simulink model "pet_integration_architecture"  (R2024a)
settings: Solver=FixedStepDiscrete  StartTime=0.0  StopTime=10.0  RelTol=1e-3
undefined symbols (not defined in the file or in its folder): D1, P
undefined symbols (not defined in the file): orig
(part 1 of 3)
settings Model: DataDictionary=pet_integration_data_dictionary.sldd  Creator=diell  LastModifiedBy=diell

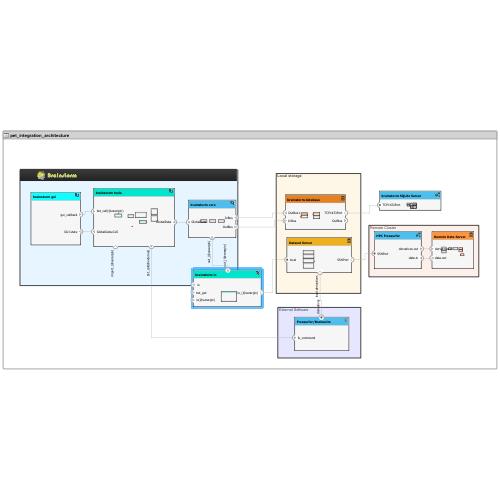
[thumbnail: Simulink's stored preview of the top-level diagram]
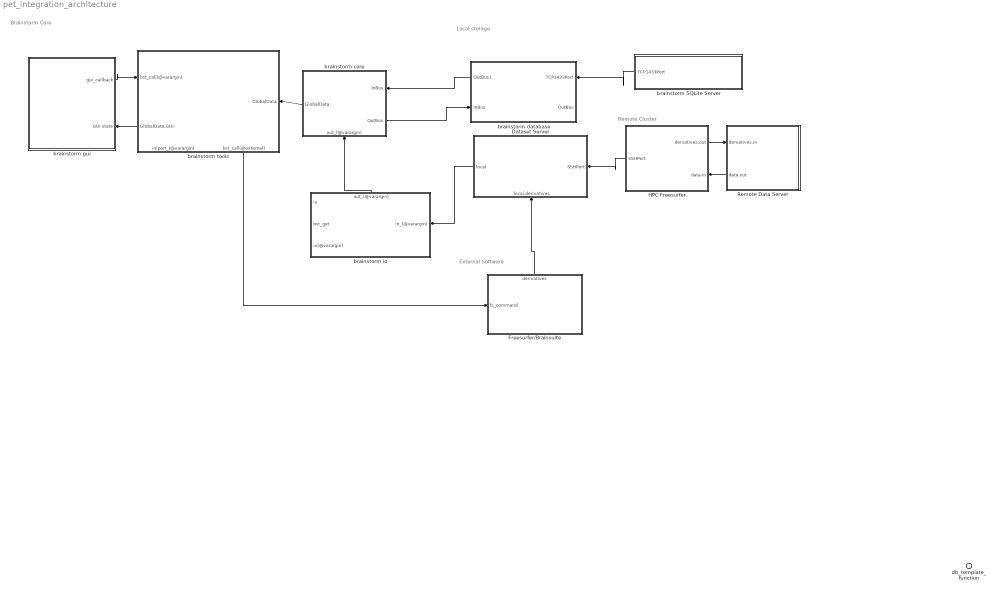
== system pet_integration_architecture ==
  note: External Software
  note: Local storage
  note: Remote Cluster
  note: Brainstorm Core
  db_template_function : Inport  OutputFunctionCall=on
  Dataset Server : Subsystem
      settings: PortSchema="{\"entries\":[{\"content\":{\"headerSize\":26,\"margin\":15,\"minimumSpacing\":25,\"sides\":[{\"content\":{\"connectorIds\":[\"Out1\"]},\"type\":\"ConnectorPlacement.EquallySpacedRectSide\",\"uuid\":\"a3539b9a-22db-4da3-b271-35b287ced3a1\"},{\"content\":{\"connectorIds\":[\"In2\"],\"side\":\"RIGHT\"},\"type\":\"ConnectorPlacement.EquallySpacedRectSide\",\"uuid\":\"72d9f298-5062-46d4-b3c5-f2fa85d7a7a6\"},{\"content\":{\"side\":\"TOP\"},\"type\":\"ConnectorPlacement.EquallySpacedRectSide\",\"uuid\":\"050469fd-3881-4b53-a813-94df038aa659\"},{\"content\":{\"connectorIds\":[\"In1\"],\"side\":\"BOTTOM\"},\"type\":\"ConnectorPlacement.EquallySpacedRectSide\",\"uuid\":\"33e80db7-af60-43f6-9c88-147327e21178\"}]},\"type\":\"ConnectorPlacement.EquallySpacedConnector\",\"uuid\":\"6db04dad-62f3-4987-a6a9-d236db4fe2a3\"}],\"packageUris\":[\"http://schema.mathworks.com/mf0/Connector/R2020b\"],\"version\":\"1.0\"}"
  Freesurfer/Brainsuite : Subsystem
      settings: PortSchema="{\"entries\":[{\"content\":{\"headerSize\":26,\"margin\":15,\"minimumSpacing\":25,\"sides\":[{\"content\":{\"connectorIds\":[\"In1\"]},\"type\":\"ConnectorPlacement.EquallySpacedRectSide\",\"uuid\":\"d9face5b-155e-4e83-95c0-d581b737b6e3\"},{\"content\":{\"side\":\"RIGHT\"},\"type\":\"ConnectorPlacement.EquallySpacedRectSide\",\"uuid\":\"f965be1f-1639-4140-b9ea-f5e9efbe4150\"},{\"content\":{\"connectorIds\":[\"Out1\"],\"side\":\"TOP\"},\"type\":\"ConnectorPlacement.EquallySpacedRectSide\",\"uuid\":\"7c9c4b2b-011c-4482-afab-b6e67025a5e2\"},{\"content\":{\"side\":\"BOTTOM\"},\"type\":\"ConnectorPlacement.EquallySpacedRectSide\",\"uuid\":\"80c85d3d-f594-4aa0-8d78-457d560265ec\"}]},\"type\":\"ConnectorPlacement.EquallySpacedConnector\",\"uuid\":\"ec963004-117d-4f22-bb00-71f35201e6e2\"}],\"packageUris\":[\"http://schema.mathworks.com/mf0/Connector/R2020b\"],\"version\":\"1.0\"}"
  HPC Freesurfer : Subsystem
      settings: PortSchema="{\"entries\":[{\"content\":{\"headerSize\":26,\"margin\":15,\"minimumSpacing\":25,\"sides\":[{\"content\":{\"connectorIds\":[\"Out1\"]},\"type\":\"ConnectorPlacement.EquallySpacedRectSide\",\"uuid\":\"d9face5b-155e-4e83-95c0-d581b737b6e3\"},{\"content\":{\"connectorIds\":[\"Out2\",\"In1\"],\"side\":\"RIGHT\"},\"type\":\"ConnectorPlacement.EquallySpacedRectSide\",\"uuid\":\"f965be1f-1639-4140-b9ea-f5e9efbe4150\"},{\"content\":{\"side\":\"TOP\"},\"type\":\"ConnectorPlacement.EquallySpacedRectSide\",\"uuid\":\"7c9c4b2b-011c-4482-afab-b6e67025a5e2\"},{\"content\":{\"side\":\"BOTTOM\"},\"type\":\"ConnectorPlacement.EquallySpacedRectSide\",\"uuid\":\"79ceda21-0cb6-4778-9565-f8bf46316a14\"}]},\"type\":\"ConnectorPlacement.EquallySpacedConnector\",\"uuid\":\"ec963004-117d-4f22-bb00-71f35201e6e2\"}],\"packageUris\":[\"http://schema.mathworks.com/mf0/Connector/R2020b\"],\"version\":\"1.0\"}"
  Remote Data Server : Subsystem
      settings: PortSchema="{\"entries\":[{\"content\":{\"headerSize\":26,\"margin\":15,\"minimumSpacing\":25,\"sides\":[{\"content\":{\"connectorIds\":[\"In1\",\"Out1\"]},\"type\":\"ConnectorPlacement.EquallySpacedRectSide\",\"uuid\":\"a3539b9a-22db-4da3-b271-35b287ced3a1\"},{\"content\":{\"side\":\"RIGHT\"},\"type\":\"ConnectorPlacement.EquallySpacedRectSide\",\"uuid\":\"72d9f298-5062-46d4-b3c5-f2fa85d7a7a6\"},{\"content\":{\"side\":\"TOP\"},\"type\":\"ConnectorPlacement.EquallySpacedRectSide\",\"uuid\":\"050469fd-3881-4b53-a813-94df038aa659\"},{\"content\":{\"side\":\"BOTTOM\"},\"type\":\"ConnectorPlacement.EquallySpacedRectSide\",\"uuid\":\"ec20b969-1eda-4ce5-89cf-082fe7652dff\"}]},\"type\":\"ConnectorPlacement.EquallySpacedConnector\",\"uuid\":\"6db04dad-62f3-4987-a6a9-d236db4fe2a3\"}],\"packageUris\":[\"http://schema.mathworks.com/mf0/Connector/R2020b\"],\"version\":\"1.0\"}"
  brainstorm SQLite Server : Subsystem
      settings: PortSchema="{\"entries\":[{\"content\":{\"headerSize\":26,\"margin\":15,\"minimumSpacing\":25,\"sides\":[{\"content\":{\"connectorIds\":[\"Out1\"]},\"type\":\"ConnectorPlacement.EquallySpacedRectSide\",\"uuid\":\"7b7365e4-3e33-4b91-9d81-29acea824425\"},{\"content\":{\"side\":\"RIGHT\"},\"type\":\"ConnectorPlacement.EquallySpacedRectSide\",\"uuid\":\"c8185be4-14fd-4b07-9d64-196ce2484816\"},{\"content\":{\"side\":\"TOP\"},\"type\":\"ConnectorPlacement.EquallySpacedRectSide\",\"uuid\":\"601e7076-ec49-4dfd-9b03-b7765df258a0\"}]},\"type\":\"ConnectorPlacement.EquallySpacedConnector\",\"uuid\":\"02951655-a26c-45d3-8145-be6034beccc3\"}],\"packageUris\":[\"http://schema.mathworks.com/mf0/Connector/R2020b\"],\"version\":\"1.0\"}"
  brainstorm core : Subsystem
      settings: PortSchema="{\"entries\":[{\"content\":{\"headerSize\":26,\"margin\":15,\"minimumSpacing\":25,\"sides\":[{\"content\":{\"connectorIds\":[\"Out2\"]},\"type\":\"ConnectorPlacement.EquallySpacedRectSide\",\"uuid\":\"f13372f0-b9c4-4d9f-b80d-b3fcffd9ebc1\"},{\"content\":{\"connectorIds\":[\"In2\",\"Out1\"],\"side\":\"RIGHT\"},\"type\":\"ConnectorPlacement.EquallySpacedRectSide\",\"uuid\":\"7a8ed507-1a09-4737-be0e-7f469c03bf31\"},{\"content\":{\"side\":\"TOP\"},\"type\":\"ConnectorPlacement.EquallySpacedRectSide\",\"uuid\":\"dcf0e4cd-c5e5-4129-a80f-1cd05790def0\"},{\"content\":{\"connectorIds\":[\"In1\"],\"side\":\"BOTTOM\"},\"type\":\"ConnectorPlacement.EquallySpacedRectSide\",\"uuid\":\"0e961a59-0b55-4a03-a714-2fdf2294d0cf\"}]},\"type\":\"ConnectorPlacement.EquallySpacedConnector\",\"uuid\":\"218acaa3-d922-4814-a102-8c4fe12f2e05\"}],\"packageUris\":[\"http://schema.mathworks.com/mf0/Connector/R2020b\"],\"version\":\"1.0\"}"
  brainstorm database : Subsystem
      settings: PortSchema="{\"entries\":[{\"content\":{\"headerSize\":26,\"margin\":15,\"minimumSpacing\":25,\"sides\":[{\"content\":{\"connectorIds\":[\"Out1\",\"In1\"]},\"type\":\"ConnectorPlacement.EquallySpacedRectSide\",\"uuid\":\"d4370dee-db71-4a38-ba8c-347b506b3053\"},{\"content\":{\"connectorIds\":[\"In2\",\"Out2\"],\"side\":\"RIGHT\"},\"type\":\"ConnectorPlacement.EquallySpacedRectSide\",\"uuid\":\"2fab9e72-f87c-493f-bacf-77c4be84942a\"},{\"content\":{\"side\":\"TOP\"},\"type\":\"ConnectorPlacement.EquallySpacedRectSide\",\"uuid\":\"3b731ab7-bbbf-4243-a071-715f3ecb33e2\"}]},\"type\":\"ConnectorPlacement.EquallySpacedConnector\",\"uuid\":\"fffe9ba9-fa34-4948-8c6e-90e3263c9a73\"}],\"packageUris\":[\"http://schema.mathworks.com/mf0/Connector/R2020b\"],\"version\":\"1.0\"}"
  brainstorm gui : Subsystem
      settings: PortSchema="{\"entries\":[{\"content\":{\"headerSize\":26,\"margin\":15,\"minimumSpacing\":25,\"sides\":[{\"content\":{},\"type\":\"ConnectorPlacement.EquallySpacedRectSide\",\"uuid\":\"d99db108-8c8a-4010-81b2-f142fbf318f5\"},{\"content\":{\"connectorIds\":[\"Out1\",\"In1\"],\"side\":\"RIGHT\"},\"type\":\"ConnectorPlacement.EquallySpacedRectSide\",\"uuid\":\"9190d96c-22e3-4cc9-a507-8f094dc67743\"},{\"content\":{\"side\":\"TOP\"},\"type\":\"ConnectorPlacement.EquallySpacedRectSide\",\"uuid\":\"08b46875-eac1-4edb-b2eb-5598dd517a75\"},{\"content\":{\"side\":\"BOTTOM\"},\"type\":\"ConnectorPlacement.EquallySpacedRectSide\",\"uuid\":\"52ff99e9-7de1-484d-abe5-5275aa089791\"}]},\"type\":\"ConnectorPlacement.EquallySpacedConnector\",\"uuid\":\"c8d2d02b-cf5a-431f-8876-22d36c8a9b33\"}],\"packageUris\":[\"http://schema.mathworks.com/mf0/Connector/R2020b\"],\"version\":\"1.0\"}"
  brainstorm io : Subsystem
      settings: PortSchema="{\"entries\":[{\"content\":{\"headerSize\":26,\"margin\":15,\"minimumSpacing\":25,\"sides\":[{\"content\":{\"connectorIds\":[\"Out1\",\"In3\",\"In2\"]},\"type\":\"ConnectorPlacement.EquallySpacedRectSide\",\"uuid\":\"d9face5b-155e-4e83-95c0-d581b737b6e3\"},{\"content\":{\"connectorIds\":[\"In1\"],\"side\":\"RIGHT\"},\"type\":\"ConnectorPlacement.EquallySpacedRectSide\",\"uuid\":\"f965be1f-1639-4140-b9ea-f5e9efbe4150\"},{\"content\":{\"connectorIds\":[\"Out2\"],\"side\":\"TOP\"},\"type\":\"ConnectorPlacement.EquallySpacedRectSide\",\"uuid\":\"7c9c4b2b-011c-4482-afab-b6e67025a5e2\"},{\"content\":{\"side\":\"BOTTOM\"},\"type\":\"ConnectorPlacement.EquallySpacedRectSide\",\"uuid\":\"6bb6967a-39ac-45ff-9bbd-a1229cc8daf0\"}]},\"type\":\"ConnectorPlacement.EquallySpacedConnector\",\"uuid\":\"ec963004-117d-4f22-bb00-71f35201e6e2\"}],\"packageUris\":[\"http://schema.mathworks.com/mf0/Connector/R2020b\"],\"version\":\"1.0\"}"
  brainstorm tools : Subsystem
      settings: PortSchema="{\"entries\":[{\"content\":{\"headerSize\":26,\"margin\":15,\"minimumSpacing\":25,\"sides\":[{\"content\":{\"connectorIds\":[\"In3\",\"Out2\"]},\"type\":\"ConnectorPlacement.EquallySpacedRectSide\",\"uuid\":\"d9face5b-155e-4e83-95c0-d581b737b6e3\"},{\"content\":{\"connectorIds\":[\"In1\"],\"side\":\"RIGHT\"},\"type\":\"ConnectorPlacement.EquallySpacedRectSide\",\"uuid\":\"f965be1f-1639-4140-b9ea-f5e9efbe4150\"},{\"content\":{\"side\":\"TOP\"},\"type\":\"ConnectorPlacement.EquallySpacedRectSide\",\"uuid\":\"7c9c4b2b-011c-4482-afab-b6e67025a5e2\"},{\"content\":{\"connectorIds\":[\"In2\",\"Out1\"],\"side\":\"BOTTOM\"},\"type\":\"ConnectorPlacement.EquallySpacedRectSide\",\"uuid\":\"7ddfacb7-8536-41fd-ae4b-23626163bd6c\"}]},\"type\":\"ConnectorPlacement.EquallySpacedConnector\",\"uuid\":\"ec963004-117d-4f22-bb00-71f35201e6e2\"}],\"packageUris\":[\"http://schema.mathworks.com/mf0/Connector/R2020b\"],\"version\":\"1.0\"}"
  wires:
  Remote Data Server/1(data.out) -> HPC Freesurfer/1(data.in)
  HPC Freesurfer/2(dervatives.out) -> Remote Data Server/1(dervatives.in)
  HPC Freesurfer/1(SSHPort) -> Dataset Server/2(SSHPort)
  brainstorm tools/2(GlobalData.GUI) -> brainstorm gui/1(GUI state)
  brainstorm gui/1(gui_callback) -> brainstorm tools/3(bst_call(@varargin))
  brainstorm tools/1(bst_call(@external)) -> Freesurfer/Brainsuite/1(fs_command)
  Freesurfer/Brainsuite/1(derivatives) -> Dataset Server/1(local.derivatives)
  brainstorm SQLite Server/1(TCP1433Port) -> brainstorm database/2(TCP1433Port)
  brainstorm core/2(GlobalData) -> brainstorm tools/1(GlobalData)
  brainstorm database/1(OutBus1) -> brainstorm core/2(InBus)
  Dataset Server/1(local) -> brainstorm io/1(in_(@varargin))
  brainstorm io/2(out_(@varargin)) -> brainstorm core/1(out_(@varargin))
  brainstorm core/1(OutBus) -> brainstorm database/1(InBus)

== system pet_integration_architecture/Dataset Server ==
  Bus Element In2 : Inport  AllowServiceAccess=on  PortName=local.derivatives
  Bus Element In1 : Inport  Port=2  AllowServiceAccess=on  PortName=SSHPort
  bids dataset : Subsystem
      settings: PortSchema="{\"entries\":[{\"content\":{\"headerSize\":26,\"margin\":15,\"minimumSpacing\":25,\"sides\":[{\"content\":{},\"type\":\"ConnectorPlacement.EquallySpacedRectSide\",\"uuid\":\"a3539b9a-22db-4da3-b271-35b287ced3a1\"},{\"content\":{\"connectorIds\":[\"Out1\"],\"side\":\"RIGHT\"},\"type\":\"ConnectorPlacement.EquallySpacedRectSide\",\"uuid\":\"72d9f298-5062-46d4-b3c5-f2fa85d7a7a6\"},{\"content\":{\"side\":\"TOP\"},\"type\":\"ConnectorPlacement.EquallySpacedRectSide\",\"uuid\":\"050469fd-3881-4b53-a813-94df038aa659\"}]},\"type\":\"ConnectorPlacement.EquallySpacedConnector\",\"uuid\":\"6db04dad-62f3-4987-a6a9-d236db4fe2a3\"}],\"packageUris\":[\"http://schema.mathworks.com/mf0/Connector/R2020b\"],\"version\":\"1.0\"}"
  brainstorm_db : Subsystem
      settings: PortSchema="{\"entries\":[{\"content\":{\"headerSize\":26,\"margin\":15,\"minimumSpacing\":25,\"sides\":[{\"content\":{},\"type\":\"ConnectorPlacement.EquallySpacedRectSide\",\"uuid\":\"a3539b9a-22db-4da3-b271-35b287ced3a1\"},{\"content\":{\"side\":\"RIGHT\"},\"type\":\"ConnectorPlacement.EquallySpacedRectSide\",\"uuid\":\"72d9f298-5062-46d4-b3c5-f2fa85d7a7a6\"},{\"content\":{\"side\":\"TOP\"},\"type\":\"ConnectorPlacement.EquallySpacedRectSide\",\"uuid\":\"050469fd-3881-4b53-a813-94df038aa659\"}]},\"type\":\"ConnectorPlacement.EquallySpacedConnector\",\"uuid\":\"6db04dad-62f3-4987-a6a9-d236db4fe2a3\"}],\"packageUris\":[\"http://schema.mathworks.com/mf0/Connector/R2020b\"],\"version\":\"1.0\"}"
  remoteConfig : Subsystem
      settings: PortSchema="{\"entries\":[{\"content\":{\"headerSize\":26,\"margin\":15,\"minimumSpacing\":25,\"sides\":[{\"content\":{},\"type\":\"ConnectorPlacement.EquallySpacedRectSide\",\"uuid\":\"a3539b9a-22db-4da3-b271-35b287ced3a1\"},{\"content\":{\"connectorIds\":[\"Out1\"],\"side\":\"RIGHT\"},\"type\":\"ConnectorPlacement.EquallySpacedRectSide\",\"uuid\":\"72d9f298-5062-46d4-b3c5-f2fa85d7a7a6\"},{\"content\":{\"side\":\"TOP\"},\"type\":\"ConnectorPlacement.EquallySpacedRectSide\",\"uuid\":\"050469fd-3881-4b53-a813-94df038aa659\"}]},\"type\":\"ConnectorPlacement.EquallySpacedConnector\",\"uuid\":\"6db04dad-62f3-4987-a6a9-d236db4fe2a3\"}],\"packageUris\":[\"http://schema.mathworks.com/mf0/Connector/R2020b\"],\"version\":\"1.0\"}"
  sourceData : Subsystem
      settings: PortSchema="{\"entries\":[{\"content\":{\"headerSize\":26,\"margin\":15,\"minimumSpacing\":25,\"sides\":[{\"content\":{},\"type\":\"ConnectorPlacement.EquallySpacedRectSide\",\"uuid\":\"1ec5f43e-86ec-4420-9dd8-c30b843d5131\"},{\"content\":{\"connectorIds\":[\"Out1\"],\"side\":\"RIGHT\"},\"type\":\"ConnectorPlacement.EquallySpacedRectSide\",\"uuid\":\"372e8174-47dc-4989-909e-f78b7a521fdc\"},{\"content\":{\"side\":\"TOP\"},\"type\":\"ConnectorPlacement.EquallySpacedRectSide\",\"uuid\":\"cc67dfee-4023-44ab-9dd9-de9f078f7d77\"},{\"content\":{\"side\":\"BOTTOM\"},\"type\":\"ConnectorPlacement.EquallySpacedRectSide\",\"uuid\":\"3cc91820-b636-4f79-822a-930cd044e5bf\"}]},\"type\":\"ConnectorPlacement.EquallySpacedConnector\",\"uuid\":\"fe3e41a6-8f67-44d2-abc6-74b481cf0464\"}],\"packageUris\":[\"http://schema.mathworks.com/mf0/Connector/R2020b\"],\"version\":\"1.0\"}"
  Bus Element Out3 : Outport  AllowServiceAccess=on  PortName=local
  wires:
  remoteConfig/1(userConfigRemote) -> ?

== system pet_integration_architecture/Freesurfer//Brainsuite ==
  Bus Element In1 : Inport  PortName=fs_command
  Brainsuite : Subsystem  VariantControl=false
      settings: PortSchema="{\"entries\":[{\"content\":{\"headerSize\":26,\"margin\":15,\"minimumSpacing\":25,\"sides\":[{\"content\":{},\"type\":\"ConnectorPlacement.EquallySpacedRectSide\",\"uuid\":\"7af8da10-a6e7-4b74-875d-43751fa02274\"},{\"content\":{\"side\":\"RIGHT\"},\"type\":\"ConnectorPlacement.EquallySpacedRectSide\",\"uuid\":\"bb27744f-ed7c-4961-9fd1-9495dcd3e5db\"},{\"content\":{\"side\":\"TOP\"},\"type\":\"ConnectorPlacement.EquallySpacedRectSide\",\"uuid\":\"a23adb5c-8f11-4285-87d6-c1c1875b2103\"}]},\"type\":\"ConnectorPlacement.EquallySpacedConnector\",\"uuid\":\"a684d927-a0c0-4e5c-9189-c4ba07d89410\"}],\"packageUris\":[\"http://schema.mathworks.com/mf0/Connector/R2020b\"],\"version\":\"1.0\"}"
  Freesurfer : Subsystem  VariantControl=true
      settings: PortSchema="{\"entries\":[{\"content\":{\"headerSize\":26,\"margin\":15,\"minimumSpacing\":25,\"sides\":[{\"content\":{},\"type\":\"ConnectorPlacement.EquallySpacedRectSide\",\"uuid\":\"7af8da10-a6e7-4b74-875d-43751fa02274\"},{\"content\":{\"connectorIds\":[\"In1\"],\"side\":\"RIGHT\"},\"type\":\"ConnectorPlacement.EquallySpacedRectSide\",\"uuid\":\"bb27744f-ed7c-4961-9fd1-9495dcd3e5db\"},{\"content\":{\"side\":\"TOP\"},\"type\":\"ConnectorPlacement.EquallySpacedRectSide\",\"uuid\":\"a23adb5c-8f11-4285-87d6-c1c1875b2103\"}]},\"type\":\"ConnectorPlacement.EquallySpacedConnector\",\"uuid\":\"a684d927-a0c0-4e5c-9189-c4ba07d89410\"}],\"packageUris\":[\"http://schema.mathworks.com/mf0/Connector/R2020b\"],\"version\":\"1.0\"}"
  Bus Element Out1 : Outport  AllowServiceAccess=on  PortName=derivatives

== system pet_integration_architecture/HPC Freesurfer ==
  Bus Element In3 : Inport  PortName=data.in
  Bus Element Out2 : Outport  AllowServiceAccess=on  PortName=SSHPort
  Bus Element Out1 : Outport  Port=2  PortName=dervatives.out

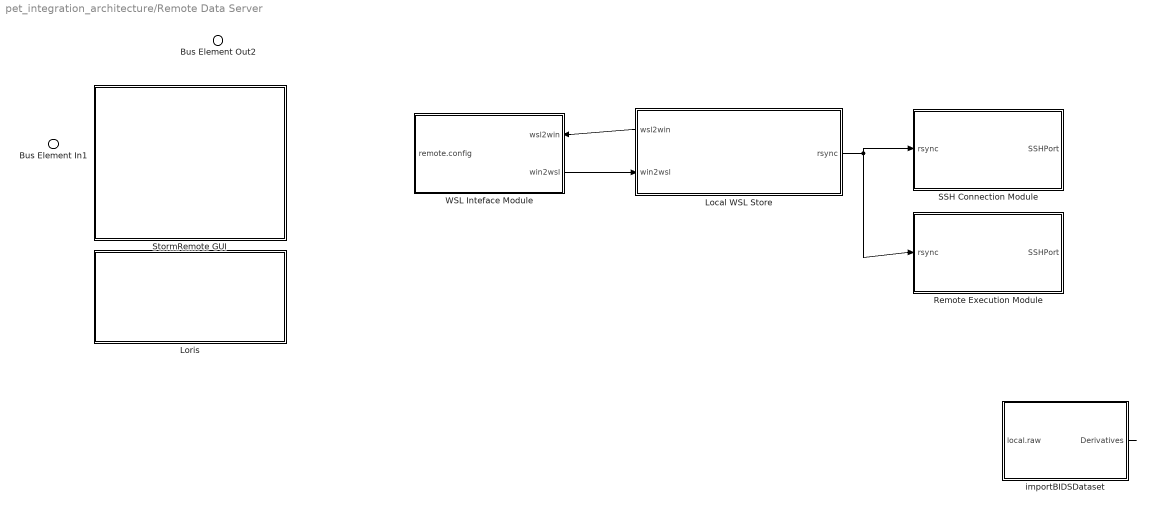
== system pet_integration_architecture/Remote Data Server ==
  Bus Element In1 : Inport  PortName=dervatives.in
  Local WSL Store : Subsystem
      settings: PortSchema="{\"entries\":[{\"content\":{\"headerSize\":26,\"margin\":15,\"minimumSpacing\":25,\"sides\":[{\"content\":{\"connectorIds\":[\"Out2\",\"In1\"]},\"type\":\"ConnectorPlacement.EquallySpacedRectSide\",\"uuid\":\"97c1e145-3d4b-49de-9739-71f2af5be190\"},{\"content\":{\"connectorIds\":[\"Out1\"],\"side\":\"RIGHT\"},\"type\":\"ConnectorPlacement.EquallySpacedRectSide\",\"uuid\":\"5a937baa-e46f-4764-8b00-75a1eb9e59b0\"},{\"content\":{\"side\":\"TOP\"},\"type\":\"ConnectorPlacement.EquallySpacedRectSide\",\"uuid\":\"83b91a39-9e34-441d-bccf-4f6b71aa9c87\"},{\"content\":{\"side\":\"BOTTOM\"},\"type\":\"ConnectorPlacement.EquallySpacedRectSide\",\"uuid\":\"5f92dfdc-6fb4-492c-a1ac-f9c6500567de\"}]},\"type\":\"ConnectorPlacement.EquallySpacedConnector\",\"uuid\":\"3f7bec2f-99ca-4d64-b419-ed6b2efa51c2\"}],\"packageUris\":[\"http://schema.mathworks.com/mf0/Connector/R2020b\"],\"version\":\"1.0\"}"
  Loris : Subsystem
      settings: PortSchema="{\"entries\":[{\"content\":{\"headerSize\":26,\"margin\":15,\"minimumSpacing\":25,\"sides\":[{\"content\":{},\"type\":\"ConnectorPlacement.EquallySpacedRectSide\",\"uuid\":\"97c1e145-3d4b-49de-9739-71f2af5be190\"},{\"content\":{\"side\":\"RIGHT\"},\"type\":\"ConnectorPlacement.EquallySpacedRectSide\",\"uuid\":\"5a937baa-e46f-4764-8b00-75a1eb9e59b0\"},{\"content\":{\"side\":\"TOP\"},\"type\":\"ConnectorPlacement.EquallySpacedRectSide\",\"uuid\":\"83b91a39-9e34-441d-bccf-4f6b71aa9c87\"}]},\"type\":\"ConnectorPlacement.EquallySpacedConnector\",\"uuid\":\"3f7bec2f-99ca-4d64-b419-ed6b2efa51c2\"}],\"packageUris\":[\"http://schema.mathworks.com/mf0/Connector/R2020b\"],\"version\":\"1.0\"}"
  Remote Execution Module : Subsystem
      settings: PortSchema="{\"entries\":[{\"content\":{\"headerSize\":26,\"margin\":15,\"minimumSpacing\":25,\"sides\":[{\"content\":{\"connectorIds\":[\"In2\"]},\"type\":\"ConnectorPlacement.EquallySpacedRectSide\",\"uuid\":\"97c1e145-3d4b-49de-9739-71f2af5be190\"},{\"content\":{\"connectorIds\":[\"In1\"],\"side\":\"RIGHT\"},\"type\":\"ConnectorPlacement.EquallySpacedRectSide\",\"uuid\":\"5a937baa-e46f-4764-8b00-75a1eb9e59b0\"},{\"content\":{\"side\":\"TOP\"},\"type\":\"ConnectorPlacement.EquallySpacedRectSide\",\"uuid\":\"83b91a39-9e34-441d-bccf-4f6b71aa9c87\"},{\"content\":{\"side\":\"BOTTOM\"},\"type\":\"ConnectorPlacement.EquallySpacedRectSide\",\"uuid\":\"3a497310-edc4-4e47-9dff-2752b4e05b5a\"}]},\"type\":\"ConnectorPlacement.EquallySpacedConnector\",\"uuid\":\"3f7bec2f-99ca-4d64-b419-ed6b2efa51c2\"}],\"packageUris\":[\"http://schema.mathworks.com/mf0/Connector/R2020b\"],\"version\":\"1.0\"}"
  SSH Connection Module : Subsystem
      settings: PortSchema="{\"entries\":[{\"content\":{\"headerSize\":26,\"margin\":15,\"minimumSpacing\":25,\"sides\":[{\"content\":{\"connectorIds\":[\"In1\"]},\"type\":\"ConnectorPlacement.EquallySpacedRectSide\",\"uuid\":\"97c1e145-3d4b-49de-9739-71f2af5be190\"},{\"content\":{\"connectorIds\":[\"In2\"],\"side\":\"RIGHT\"},\"type\":\"ConnectorPlacement.EquallySpacedRectSide\",\"uuid\":\"5a937baa-e46f-4764-8b00-75a1eb9e59b0\"},{\"content\":{\"side\":\"TOP\"},\"type\":\"ConnectorPlacement.EquallySpacedRectSide\",\"uuid\":\"83b91a39-9e34-441d-bccf-4f6b71aa9c87\"},{\"content\":{\"side\":\"BOTTOM\"},\"type\":\"ConnectorPlacement.EquallySpacedRectSide\",\"uuid\":\"1fa9e83f-f2ec-4121-bd0c-70c9fe2d9333\"}]},\"type\":\"ConnectorPlacement.EquallySpacedConnector\",\"uuid\":\"3f7bec2f-99ca-4d64-b419-ed6b2efa51c2\"}],\"packageUris\":[\"http://schema.mathworks.com/mf0/Connector/R2020b\"],\"version\":\"1.0\"}"
  StormRemote GUI : Subsystem
      settings: PortSchema="{\"entries\":[{\"content\":{\"headerSize\":26,\"margin\":15,\"minimumSpacing\":25,\"sides\":[{\"content\":{},\"type\":\"ConnectorPlacement.EquallySpacedRectSide\",\"uuid\":\"97c1e145-3d4b-49de-9739-71f2af5be190\"},{\"content\":{\"side\":\"RIGHT\"},\"type\":\"ConnectorPlacement.EquallySpacedRectSide\",\"uuid\":\"5a937baa-e46f-4764-8b00-75a1eb9e59b0\"},{\"content\":{\"side\":\"TOP\"},\"type\":\"ConnectorPlacement.EquallySpacedRectSide\",\"uuid\":\"83b91a39-9e34-441d-bccf-4f6b71aa9c87\"}]},\"type\":\"ConnectorPlacement.EquallySpacedConnector\",\"uuid\":\"3f7bec2f-99ca-4d64-b419-ed6b2efa51c2\"}],\"packageUris\":[\"http://schema.mathworks.com/mf0/Connector/R2020b\"],\"version\":\"1.0\"}"
  WSL Inteface Module : Subsystem
      settings: PortSchema="{\"entries\":[{\"content\":{\"headerSize\":26,\"margin\":15,\"minimumSpacing\":25,\"sides\":[{\"content\":{\"connectorIds\":[\"In2\"]},\"type\":\"ConnectorPlacement.EquallySpacedRectSide\",\"uuid\":\"97c1e145-3d4b-49de-9739-71f2af5be190\"},{\"content\":{\"connectorIds\":[\"In1\",\"Out1\"],\"side\":\"RIGHT\"},\"type\":\"ConnectorPlacement.EquallySpacedRectSide\",\"uuid\":\"5a937baa-e46f-4764-8b00-75a1eb9e59b0\"},{\"content\":{\"side\":\"TOP\"},\"type\":\"ConnectorPlacement.EquallySpacedRectSide\",\"uuid\":\"83b91a39-9e34-441d-bccf-4f6b71aa9c87\"}]},\"type\":\"ConnectorPlacement.EquallySpacedConnector\",\"uuid\":\"3f7bec2f-99ca-4d64-b419-ed6b2efa51c2\"}],\"packageUris\":[\"http://schema.mathworks.com/mf0/Connector/R2020b\"],\"version\":\"1.0\"}"
  importBIDSDataset : Subsystem
      settings: PortSchema="{\"entries\":[{\"content\":{\"headerSize\":26,\"margin\":15,\"minimumSpacing\":25,\"sides\":[{\"content\":{\"connectorIds\":[\"In1\"]},\"type\":\"ConnectorPlacement.EquallySpacedRectSide\",\"uuid\":\"2137c5ed-fa53-439b-a426-32e4a43756b1\"},{\"content\":{\"connectorIds\":[\"Out1\"],\"side\":\"RIGHT\"},\"type\":\"ConnectorPlacement.EquallySpacedRectSide\",\"uuid\":\"48b1940f-4cec-47e5-85cc-9407b18f8963\"},{\"content\":{\"side\":\"TOP\"},\"type\":\"ConnectorPlacement.EquallySpacedRectSide\",\"uuid\":\"d0a26462-f6c6-4c35-8d3a-db787c6ff794\"}]},\"type\":\"ConnectorPlacement.EquallySpacedConnector\",\"uuid\":\"bc57efb8-a3db-4139-b3a9-b2d63151e796\"}],\"packageUris\":[\"http://schema.mathworks.com/mf0/Connector/R2020b\"],\"version\":\"1.0\"}"
  Bus Element Out2 : Outport  PortName=data.out
  wires:
  WSL Inteface Module/1(win2wsl) -> Local WSL Store/1(win2wsl)
  ? -> WSL Inteface Module/2(remote.config)
  Local WSL Store/2(wsl2win) -> WSL Inteface Module/1(wsl2win)
  ? -> SSH Connection Module/2(SSHPort)
  Local WSL Store/1(rsync) -> Remote Execution Module/2(rsync), SSH Connection Module/1(rsync)
  ? -> Remote Execution Module/1(SSHPort)
  ? -> importBIDSDataset/1(local.raw)
  importBIDSDataset/1(Derivatives) -> ?

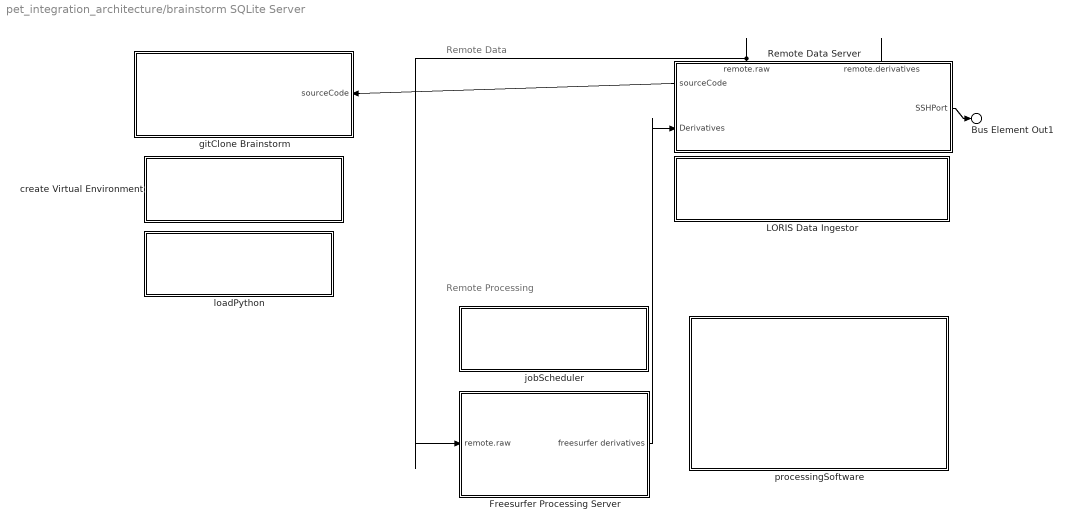
== system pet_integration_architecture/brainstorm SQLite Server ==
  note: Remote Data
  note: Remote Processing
  Freesurfer Processing Server : Subsystem
      settings: PortSchema="{\"entries\":[{\"content\":{\"headerSize\":26,\"margin\":15,\"minimumSpacing\":25,\"sides\":[{\"content\":{\"connectorIds\":[\"In1\"]},\"type\":\"ConnectorPlacement.EquallySpacedRectSide\",\"uuid\":\"d99db108-8c8a-4010-81b2-f142fbf318f5\"},{\"content\":{\"connectorIds\":[\"Out1\"],\"side\":\"RIGHT\"},\"type\":\"ConnectorPlacement.EquallySpacedRectSide\",\"uuid\":\"9190d96c-22e3-4cc9-a507-8f094dc67743\"},{\"content\":{\"side\":\"TOP\"},\"type\":\"ConnectorPlacement.EquallySpacedRectSide\",\"uuid\":\"08b46875-eac1-4edb-b2eb-5598dd517a75\"},{\"content\":{\"side\":\"BOTTOM\"},\"type\":\"ConnectorPlacement.EquallySpacedRectSide\",\"uuid\":\"ace7fe11-fb05-49db-a7ee-0fa9beffa30a\"}]},\"type\":\"ConnectorPlacement.EquallySpacedConnector\",\"uuid\":\"c8d2d02b-cf5a-431f-8876-22d36c8a9b33\"}],\"packageUris\":[\"http://schema.mathworks.com/mf0/Connector/R2020b\"],\"version\":\"1.0\"}"
  LORIS Data Ingestor : Subsystem
      settings: PortSchema="{\"entries\":[{\"content\":{\"headerSize\":26,\"margin\":15,\"minimumSpacing\":25,\"sides\":[{\"content\":{},\"type\":\"ConnectorPlacement.EquallySpacedRectSide\",\"uuid\":\"a3539b9a-22db-4da3-b271-35b287ced3a1\"},{\"content\":{\"side\":\"RIGHT\"},\"type\":\"ConnectorPlacement.EquallySpacedRectSide\",\"uuid\":\"72d9f298-5062-46d4-b3c5-f2fa85d7a7a6\"},{\"content\":{\"side\":\"TOP\"},\"type\":\"ConnectorPlacement.EquallySpacedRectSide\",\"uuid\":\"050469fd-3881-4b53-a813-94df038aa659\"}]},\"type\":\"ConnectorPlacement.EquallySpacedConnector\",\"uuid\":\"6db04dad-62f3-4987-a6a9-d236db4fe2a3\"}],\"packageUris\":[\"http://schema.mathworks.com/mf0/Connector/R2020b\"],\"version\":\"1.0\"}"
  Remote Data Server : Subsystem
      settings: PortSchema="{\"entries\":[{\"content\":{\"headerSize\":26,\"margin\":15,\"minimumSpacing\":25,\"sides\":[{\"content\":{\"connectorIds\":[\"Out1\",\"In1\"]},\"type\":\"ConnectorPlacement.EquallySpacedRectSide\",\"uuid\":\"d99db108-8c8a-4010-81b2-f142fbf318f5\"},{\"content\":{\"connectorIds\":[\"Out2\"],\"side\":\"RIGHT\"},\"type\":\"ConnectorPlacement.EquallySpacedRectSide\",\"uuid\":\"9190d96c-22e3-4cc9-a507-8f094dc67743\"},{\"content\":{\"connectorIds\":[\"Out3\",\"Out4\"],\"side\":\"TOP\"},\"type\":\"ConnectorPlacement.EquallySpacedRectSide\",\"uuid\":\"08b46875-eac1-4edb-b2eb-5598dd517a75\"},{\"content\":{\"side\":\"BOTTOM\"},\"type\":\"ConnectorPlacement.EquallySpacedRectSide\",\"uuid\":\"000c332a-c8c2-4c2b-a822-ffa253837487\"}]},\"type\":\"ConnectorPlacement.EquallySpacedConnector\",\"uuid\":\"c8d2d02b-cf5a-431f-8876-22d36c8a9b33\"}],\"packageUris\":[\"http://schema.mathworks.com/mf0/Connector/R2020b\"],\"version\":\"1.0\"}"
  create Virtual Environment : Subsystem
      settings: PortSchema="{\"entries\":[{\"content\":{\"headerSize\":26,\"margin\":15,\"minimumSpacing\":25,\"sides\":[{\"content\":{},\"type\":\"ConnectorPlacement.EquallySpacedRectSide\",\"uuid\":\"a3539b9a-22db-4da3-b271-35b287ced3a1\"},{\"content\":{\"side\":\"RIGHT\"},\"type\":\"ConnectorPlacement.EquallySpacedRectSide\",\"uuid\":\"72d9f298-5062-46d4-b3c5-f2fa85d7a7a6\"},{\"content\":{\"side\":\"TOP\"},\"type\":\"ConnectorPlacement.EquallySpacedRectSide\",\"uuid\":\"050469fd-3881-4b53-a813-94df038aa659\"}]},\"type\":\"ConnectorPlacement.EquallySpacedConnector\",\"uuid\":\"6db04dad-62f3-4987-a6a9-d236db4fe2a3\"}],\"packageUris\":[\"http://schema.mathworks.com/mf0/Connector/R2020b\"],\"version\":\"1.0\"}"
  gitClone Brainstorm : Subsystem
      settings: PortSchema="{\"entries\":[{\"content\":{\"headerSize\":26,\"margin\":15,\"minimumSpacing\":25,\"sides\":[{\"content\":{},\"type\":\"ConnectorPlacement.EquallySpacedRectSide\",\"uuid\":\"a3539b9a-22db-4da3-b271-35b287ced3a1\"},{\"content\":{\"connectorIds\":[\"In1\"],\"side\":\"RIGHT\"},\"type\":\"ConnectorPlacement.EquallySpacedRectSide\",\"uuid\":\"72d9f298-5062-46d4-b3c5-f2fa85d7a7a6\"},{\"content\":{\"side\":\"TOP\"},\"type\":\"ConnectorPlacement.EquallySpacedRectSide\",\"uuid\":\"050469fd-3881-4b53-a813-94df038aa659\"}]},\"type\":\"ConnectorPlacement.EquallySpacedConnector\",\"uuid\":\"6db04dad-62f3-4987-a6a9-d236db4fe2a3\"}],\"packageUris\":[\"http://schema.mathworks.com/mf0/Connector/R2020b\"],\"version\":\"1.0\"}"
  jobScheduler : Subsystem
      settings: PortSchema="{\"entries\":[{\"content\":{\"headerSize\":26,\"margin\":15,\"minimumSpacing\":25,\"sides\":[{\"content\":{},\"type\":\"ConnectorPlacement.EquallySpacedRectSide\",\"uuid\":\"a3539b9a-22db-4da3-b271-35b287ced3a1\"},{\"content\":{\"side\":\"RIGHT\"},\"type\":\"ConnectorPlacement.EquallySpacedRectSide\",\"uuid\":\"72d9f298-5062-46d4-b3c5-f2fa85d7a7a6\"},{\"content\":{\"side\":\"TOP\"},\"type\":\"ConnectorPlacement.EquallySpacedRectSide\",\"uuid\":\"050469fd-3881-4b53-a813-94df038aa659\"}]},\"type\":\"ConnectorPlacement.EquallySpacedConnector\",\"uuid\":\"6db04dad-62f3-4987-a6a9-d236db4fe2a3\"}],\"packageUris\":[\"http://schema.mathworks.com/mf0/Connector/R2020b\"],\"version\":\"1.0\"}"
  loadPython : Subsystem
      settings: PortSchema="{\"entries\":[{\"content\":{\"headerSize\":26,\"margin\":15,\"minimumSpacing\":25,\"sides\":[{\"content\":{},\"type\":\"ConnectorPlacement.EquallySpacedRectSide\",\"uuid\":\"a3539b9a-22db-4da3-b271-35b287ced3a1\"},{\"content\":{\"side\":\"RIGHT\"},\"type\":\"ConnectorPlacement.EquallySpacedRectSide\",\"uuid\":\"72d9f298-5062-46d4-b3c5-f2fa85d7a7a6\"},{\"content\":{\"side\":\"TOP\"},\"type\":\"ConnectorPlacement.EquallySpacedRectSide\",\"uuid\":\"050469fd-3881-4b53-a813-94df038aa659\"}]},\"type\":\"ConnectorPlacement.EquallySpacedConnector\",\"uuid\":\"6db04dad-62f3-4987-a6a9-d236db4fe2a3\"}],\"packageUris\":[\"http://schema.mathworks.com/mf0/Connector/R2020b\"],\"version\":\"1.0\"}"
  processingSoftware : Subsystem
      settings: PortSchema="{\"entries\":[{\"content\":{\"headerSize\":26,\"margin\":15,\"minimumSpacing\":25,\"sides\":[{\"content\":{},\"type\":\"ConnectorPlacement.EquallySpacedRectSide\",\"uuid\":\"a3539b9a-22db-4da3-b271-35b287ced3a1\"},{\"content\":{\"side\":\"RIGHT\"},\"type\":\"ConnectorPlacement.EquallySpacedRectSide\",\"uuid\":\"72d9f298-5062-46d4-b3c5-f2fa85d7a7a6\"},{\"content\":{\"side\":\"TOP\"},\"type\":\"ConnectorPlacement.EquallySpacedRectSide\",\"uuid\":\"050469fd-3881-4b53-a813-94df038aa659\"}]},\"type\":\"ConnectorPlacement.EquallySpacedConnector\",\"uuid\":\"6db04dad-62f3-4987-a6a9-d236db4fe2a3\"}],\"packageUris\":[\"http://schema.mathworks.com/mf0/Connector/R2020b\"],\"version\":\"1.0\"}"
  Bus Element Out1 : Outport  AllowServiceAccess=on  PortName=TCP1433Port
  wires:
  Remote Data Server/3(remote.raw) -> Freesurfer Processing Server/1(remote.raw)
  Freesurfer Processing Server/1(freesurfer derivatives) -> Remote Data Server/1(Derivatives)
  Remote Data Server/4(remote.derivatives) -> ?
  Remote Data Server/2(SSHPort) -> Bus Element Out1/1
  Remote Data Server/1(sourceCode) -> gitClone Brainstorm/1(sourceCode)

== system pet_integration_architecture/brainstorm core ==
  Bus Element In2 : Inport  PortName=out_(@varargin)
  Bus Element In1 : Inport  Port=2  PortName=InBus
  bst_get : Subsystem
      settings: PortSchema="{\"entries\":[{\"content\":{\"headerSize\":26,\"margin\":15,\"minimumSpacing\":25,\"sides\":[{\"content\":{},\"type\":\"ConnectorPlacement.EquallySpacedRectSide\",\"uuid\":\"f13372f0-b9c4-4d9f-b80d-b3fcffd9ebc1\"},{\"content\":{\"side\":\"RIGHT\"},\"type\":\"ConnectorPlacement.EquallySpacedRectSide\",\"uuid\":\"7a8ed507-1a09-4737-be0e-7f469c03bf31\"},{\"content\":{\"side\":\"TOP\"},\"type\":\"ConnectorPlacement.EquallySpacedRectSide\",\"uuid\":\"dcf0e4cd-c5e5-4129-a80f-1cd05790def0\"}]},\"type\":\"ConnectorPlacement.EquallySpacedConnector\",\"uuid\":\"218acaa3-d922-4814-a102-8c4fe12f2e05\"}],\"packageUris\":[\"http://schema.mathworks.com/mf0/Connector/R2020b\"],\"version\":\"1.0\"}"
  bst_set : Subsystem
      settings: PortSchema="{\"entries\":[{\"content\":{\"headerSize\":26,\"margin\":15,\"minimumSpacing\":25,\"sides\":[{\"content\":{},\"type\":\"ConnectorPlacement.EquallySpacedRectSide\",\"uuid\":\"f13372f0-b9c4-4d9f-b80d-b3fcffd9ebc1\"},{\"content\":{\"side\":\"RIGHT\"},\"type\":\"ConnectorPlacement.EquallySpacedRectSide\",\"uuid\":\"7a8ed507-1a09-4737-be0e-7f469c03bf31\"},{\"content\":{\"side\":\"TOP\"},\"type\":\"ConnectorPlacement.EquallySpacedRectSide\",\"uuid\":\"dcf0e4cd-c5e5-4129-a80f-1cd05790def0\"}]},\"type\":\"ConnectorPlacement.EquallySpacedConnector\",\"uuid\":\"218acaa3-d922-4814-a102-8c4fe12f2e05\"}],\"packageUris\":[\"http://schema.mathworks.com/mf0/Connector/R2020b\"],\"version\":\"1.0\"}"
  db_template : ModelReference  ModelNameDialog=db_template_model  SimulationMode=Normal  ScheduleRates=on  ModelEventPortInfo=P:D1[-2][0][0]  ModelReferenceVersion=1.11
      settings: PortSchema="{\"entries\":[{\"content\":{\"headerSize\":38,\"margin\":15,\"minimumSpacing\":25,\"sides\":[{\"content\":{\"connectorIds\":[\"In1\"]},\"type\":\"ConnectorPlacement.EquallySpacedRectSide\",\"uuid\":\"f13372f0-b9c4-4d9f-b80d-b3fcffd9ebc1\"},{\"content\":{\"connectorIds\":[\"Out1\"],\"side\":\"RIGHT\"},\"type\":\"ConnectorPlacement.EquallySpacedRectSide\",\"uuid\":\"7a8ed507-1a09-4737-be0e-7f469c03bf31\"},{\"content\":{\"side\":\"TOP\"},\"type\":\"ConnectorPlacement.EquallySpacedRectSide\",\"uuid\":\"dcf0e4cd-c5e5-4129-a80f-1cd05790def0\"},{\"content\":{\"connectorIds\":[\"In2\"],\"side\":\"HIDDEN\"},\"type\":\"ConnectorPlacement.EquallySpacedRectSide\",\"uuid\":\"43ebb3c1-16d1-4ff0-922d-5285315156b5\"}]},\"type\":\"ConnectorPlacement.EquallySpacedConnector\",\"uuid\":\"218acaa3-d922-4814-a102-8c4fe12f2e05\"}],\"packageUris\":[\"http://schema.mathworks.com/mf0/Connector/R2020b\"],\"version\":\"1.0\"}"
  Bus Element Out2 : Outport  PortName=OutBus
  Bus Element Out1 : Outport  Port=2  PortName=GlobalData

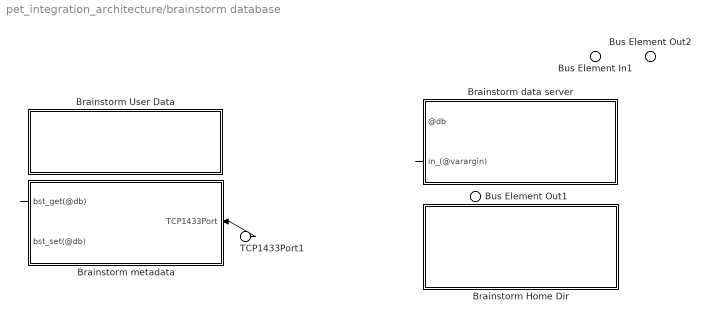
== system pet_integration_architecture/brainstorm database ==
  Bus Element In1 : Inport  PortName=InBus
  TCP1433Port1 : Inport  Port=2  AllowServiceAccess=on  PortName=TCP1433Port
  Brainstorm Home Dir : Subsystem
      settings: PortSchema="{\"entries\":[{\"content\":{\"headerSize\":26,\"margin\":15,\"minimumSpacing\":25,\"sides\":[{\"content\":{},\"type\":\"ConnectorPlacement.EquallySpacedRectSide\",\"uuid\":\"f13372f0-b9c4-4d9f-b80d-b3fcffd9ebc1\"},{\"content\":{\"side\":\"RIGHT\"},\"type\":\"ConnectorPlacement.EquallySpacedRectSide\",\"uuid\":\"7a8ed507-1a09-4737-be0e-7f469c03bf31\"},{\"content\":{\"side\":\"TOP\"},\"type\":\"ConnectorPlacement.EquallySpacedRectSide\",\"uuid\":\"dcf0e4cd-c5e5-4129-a80f-1cd05790def0\"}]},\"type\":\"ConnectorPlacement.EquallySpacedConnector\",\"uuid\":\"218acaa3-d922-4814-a102-8c4fe12f2e05\"}],\"packageUris\":[\"http://schema.mathworks.com/mf0/Connector/R2020b\"],\"version\":\"1.0\"}"
  "Brainstorm User Data " : Subsystem
      settings: PortSchema="{\"entries\":[{\"content\":{\"headerSize\":26,\"margin\":15,\"minimumSpacing\":25,\"sides\":[{\"content\":{},\"type\":\"ConnectorPlacement.EquallySpacedRectSide\",\"uuid\":\"f13372f0-b9c4-4d9f-b80d-b3fcffd9ebc1\"},{\"content\":{\"side\":\"RIGHT\"},\"type\":\"ConnectorPlacement.EquallySpacedRectSide\",\"uuid\":\"7a8ed507-1a09-4737-be0e-7f469c03bf31\"},{\"content\":{\"side\":\"TOP\"},\"type\":\"ConnectorPlacement.EquallySpacedRectSide\",\"uuid\":\"dcf0e4cd-c5e5-4129-a80f-1cd05790def0\"}]},\"type\":\"ConnectorPlacement.EquallySpacedConnector\",\"uuid\":\"218acaa3-d922-4814-a102-8c4fe12f2e05\"}],\"packageUris\":[\"http://schema.mathworks.com/mf0/Connector/R2020b\"],\"version\":\"1.0\"}"
  Brainstorm data server : Subsystem
      settings: PortSchema="{\"entries\":[{\"content\":{\"headerSize\":26,\"margin\":15,\"minimumSpacing\":25,\"sides\":[{\"content\":{\"connectorIds\":[\"In1\",\"Out1\"]},\"type\":\"ConnectorPlacement.EquallySpacedRectSide\",\"uuid\":\"9dc41937-0423-4f0d-95de-6a11876dea92\"},{\"content\":{\"side\":\"RIGHT\"},\"type\":\"ConnectorPlacement.EquallySpacedRectSide\",\"uuid\":\"a760f902-bb88-44c6-9e15-f93a06bbb22c\"},{\"content\":{\"side\":\"TOP\"},\"type\":\"ConnectorPlacement.EquallySpacedRectSide\",\"uuid\":\"a141426c-a194-4d5c-ba1a-f6f4f49c40a6\"},{\"content\":{\"side\":\"BOTTOM\"},\"type\":\"ConnectorPlacement.EquallySpacedRectSide\",\"uuid\":\"911cff6f-b234-4e66-a2d4-fe42114051d6\"}]},\"type\":\"ConnectorPlacement.EquallySpacedConnector\",\"uuid\":\"ec924d27-401c-47e0-a07a-aece678b254f\"}],\"packageUris\":[\"http://schema.mathworks.com/mf0/Connector/R2020b\"],\"version\":\"1.0\"}"
  "Brainstorm metadata " : Subsystem
      settings: PortSchema="{\"entries\":[{\"content\":{\"headerSize\":26,\"margin\":15,\"minimumSpacing\":25,\"sides\":[{\"content\":{\"connectorIds\":[\"Out1\",\"In1\"]},\"type\":\"ConnectorPlacement.EquallySpacedRectSide\",\"uuid\":\"9dc41937-0423-4f0d-95de-6a11876dea92\"},{\"content\":{\"connectorIds\":[\"In2\"],\"side\":\"RIGHT\"},\"type\":\"ConnectorPlacement.EquallySpacedRectSide\",\"uuid\":\"a760f902-bb88-44c6-9e15-f93a06bbb22c\"},{\"content\":{\"side\":\"TOP\"},\"type\":\"ConnectorPlacement.EquallySpacedRectSide\",\"uuid\":\"a141426c-a194-4d5c-ba1a-f6f4f49c40a6\"},{\"content\":{\"side\":\"BOTTOM\"},\"type\":\"ConnectorPlacement.EquallySpacedRectSide\",\"uuid\":\"ac179f26-87f4-4829-a285-b5f71d76bb12\"}]},\"type\":\"ConnectorPlacement.EquallySpacedConnector\",\"uuid\":\"ec924d27-401c-47e0-a07a-aece678b254f\"}],\"packageUris\":[\"http://schema.mathworks.com/mf0/Connector/R2020b\"],\"version\":\"1.0\"}"
  Bus Element Out2 : Outport  PortName=OutBus1
  Bus Element Out1 : Outport  Port=2  PortName=OutBus
  wires:
  TCP1433Port1/1 -> "Brainstorm metadata "/2(TCP1433Port)
  ? -> "Brainstorm metadata "/1(bst_set(@db))
  ? -> Brainstorm data server/1(@db)
  "Brainstorm metadata "/1(bst_get(@db)) -> ?
  Brainstorm data server/1(in_(@varargin)) -> ?

== system pet_integration_architecture/brainstorm gui ==
  Bus Element In1 : Inport  PortName=GUI state
  gui_component ('Import PET') : Subsystem
      settings: PortSchema="{\"entries\":[{\"content\":{\"headerSize\":26,\"margin\":15,\"minimumSpacing\":25,\"sides\":[{\"content\":{},\"type\":\"ConnectorPlacement.EquallySpacedRectSide\",\"uuid\":\"e452b68a-48a0-46a4-9e6b-6a7ab63d76ba\"},{\"content\":{\"connectorIds\":[\"Out1\"],\"side\":\"RIGHT\"},\"type\":\"ConnectorPlacement.EquallySpacedRectSide\",\"uuid\":\"bfc23a96-7562-4108-a377-c6d682106293\"},{\"content\":{\"side\":\"TOP\"},\"type\":\"ConnectorPlacement.EquallySpacedRectSide\",\"uuid\":\"898805eb-9365-4e37-9830-3cdbb7191da7\"}]},\"type\":\"ConnectorPlacement.EquallySpacedConnector\",\"uuid\":\"9a83eb3e-c81f-4df4-a7ca-e8a116b52f55\"}],\"packageUris\":[\"http://schema.mathworks.com/mf0/Connector/R2020b\"],\"version\":\"1.0\"}"
  Bus Element Out4 : Outport  PortName=gui_callback
  wires:
  gui_component ('Import PET')/1(gui_callback) -> Bus Element Out4/1

== system pet_integration_architecture/brainstorm io ==
  Bus Element In1 : Inport  AllowServiceAccess=on  PortName=in_(@varargin)
  Bus Element In3 : Inport  Port=2  PortName=io(@varargin)
  In Bus Element1 : Inport  Port=3  PortName=bst_get
  import_pet : Subsystem
      settings: PortSchema="{\"entries\":[{\"content\":{\"headerSize\":26,\"margin\":15,\"minimumSpacing\":25,\"sides\":[{\"content\":{\"connectorIds\":[\"In1\"]},\"type\":\"ConnectorPlacement.EquallySpacedRectSide\",\"uuid\":\"e452b68a-48a0-46a4-9e6b-6a7ab63d76ba\"},{\"content\":{\"connectorIds\":[\"Out1\"],\"side\":\"RIGHT\"},\"type\":\"ConnectorPlacement.EquallySpacedRectSide\",\"uuid\":\"bfc23a96-7562-4108-a377-c6d682106293\"},{\"content\":{\"side\":\"TOP\"},\"type\":\"ConnectorPlacement.EquallySpacedRectSide\",\"uuid\":\"898805eb-9365-4e37-9830-3cdbb7191da7\"},{\"content\":{\"connectorIds\":[\"In2\"],\"side\":\"BOTTOM\"},\"type\":\"ConnectorPlacement.EquallySpacedRectSide\",\"uuid\":\"20ed5406-47d9-41fc-b360-c996f9e858c0\"}]},\"type\":\"ConnectorPlacement.EquallySpacedConnector\",\"uuid\":\"9a83eb3e-c81f-4df4-a7ca-e8a116b52f55\"}],\"packageUris\":[\"http://schema.mathworks.com/mf0/Connector/R2020b\"],\"version\":\"1.0\"}"
  Bus Element Out2 : Outport  PortName=io
  Bus Element Out1 : Outport  Port=2  PortName=out_(@varargin)

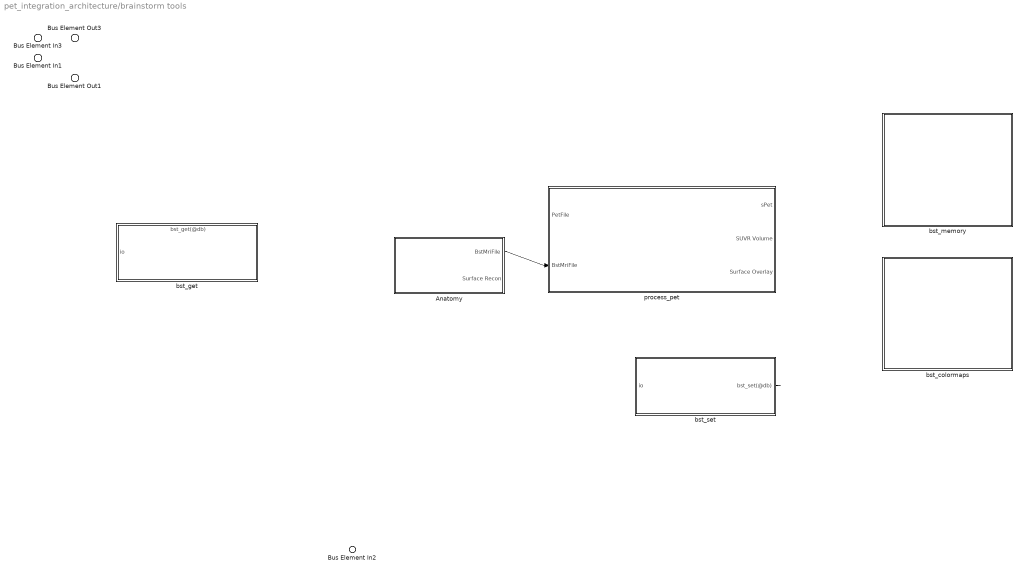
== system pet_integration_architecture/brainstorm tools ==
  Bus Element In3 : Inport  PortName=GlobalData
  Bus Element In2 : Inport  Port=2  AllowServiceAccess=on  PortName=import_(@varargin)
  Bus Element In1 : Inport  Port=3  PortName=bst_call(@varargin)
  Anatomy : Subsystem
      settings: PortSchema="{\"entries\":[{\"content\":{\"headerSize\":26,\"margin\":15,\"minimumSpacing\":25,\"sides\":[{\"content\":{},\"type\":\"ConnectorPlacement.EquallySpacedRectSide\",\"uuid\":\"d99db108-8c8a-4010-81b2-f142fbf318f5\"},{\"content\":{\"connectorIds\":[\"Out2\",\"Out1\"],\"side\":\"RIGHT\"},\"type\":\"ConnectorPlacement.EquallySpacedRectSide\",\"uuid\":\"9190d96c-22e3-4cc9-a507-8f094dc67743\"},{\"content\":{\"side\":\"TOP\"},\"type\":\"ConnectorPlacement.EquallySpacedRectSide\",\"uuid\":\"08b46875-eac1-4edb-b2eb-5598dd517a75\"}]},\"type\":\"ConnectorPlacement.EquallySpacedConnector\",\"uuid\":\"c8d2d02b-cf5a-431f-8876-22d36c8a9b33\"}],\"packageUris\":[\"http://schema.mathworks.com/mf0/Connector/R2020b\"],\"version\":\"1.0\"}"
  bst_colormaps : Subsystem
      settings: PortSchema="{\"entries\":[{\"content\":{\"headerSize\":26,\"margin\":15,\"minimumSpacing\":25,\"sides\":[{\"content\":{},\"type\":\"ConnectorPlacement.EquallySpacedRectSide\",\"uuid\":\"f13372f0-b9c4-4d9f-b80d-b3fcffd9ebc1\"},{\"content\":{\"side\":\"RIGHT\"},\"type\":\"ConnectorPlacement.EquallySpacedRectSide\",\"uuid\":\"7a8ed507-1a09-4737-be0e-7f469c03bf31\"},{\"content\":{\"side\":\"TOP\"},\"type\":\"ConnectorPlacement.EquallySpacedRectSide\",\"uuid\":\"dcf0e4cd-c5e5-4129-a80f-1cd05790def0\"}]},\"type\":\"ConnectorPlacement.EquallySpacedConnector\",\"uuid\":\"218acaa3-d922-4814-a102-8c4fe12f2e05\"}],\"packageUris\":[\"http://schema.mathworks.com/mf0/Connector/R2020b\"],\"version\":\"1.0\"}"
  bst_get : Subsystem
      settings: PortSchema="{\"entries\":[{\"content\":{\"headerSize\":26,\"margin\":15,\"minimumSpacing\":25,\"sides\":[{\"content\":{\"connectorIds\":[\"Out1\"]},\"type\":\"ConnectorPlacement.EquallySpacedRectSide\",\"uuid\":\"b493315f-c6c8-42ab-8e4d-b8fe240af9dd\"},{\"content\":{\"side\":\"RIGHT\"},\"type\":\"ConnectorPlacement.EquallySpacedRectSide\",\"uuid\":\"94c0e42b-c474-4070-8a16-a26ac22942e6\"},{\"content\":{\"connectorIds\":[\"In1\"],\"side\":\"TOP\"},\"type\":\"ConnectorPlacement.EquallySpacedRectSide\",\"uuid\":\"f9bc43e9-5c3a-451c-b434-9225c48927cc\"},{\"content\":{\"side\":\"BOTTOM\"},\"type\":\"ConnectorPlacement.EquallySpacedRectSide\",\"uuid\":\"561f7f4a-dd6b-4ca4-b56e-b79619c3d586\"}]},\"type\":\"ConnectorPlacement.EquallySpacedConnector\",\"uuid\":\"067458af-ee7c-44e6-8802-98d558b25815\"}],\"packageUris\":[\"http://schema.mathworks.com/mf0/Connector/R2020b\"],\"version\":\"1.0\"}"
  bst_memory : Subsystem
      settings: PortSchema="{\"entries\":[{\"content\":{\"headerSize\":26,\"margin\":15,\"minimumSpacing\":25,\"sides\":[{\"content\":{},\"type\":\"ConnectorPlacement.EquallySpacedRectSide\",\"uuid\":\"f13372f0-b9c4-4d9f-b80d-b3fcffd9ebc1\"},{\"content\":{\"side\":\"RIGHT\"},\"type\":\"ConnectorPlacement.EquallySpacedRectSide\",\"uuid\":\"7a8ed507-1a09-4737-be0e-7f469c03bf31\"},{\"content\":{\"side\":\"TOP\"},\"type\":\"ConnectorPlacement.EquallySpacedRectSide\",\"uuid\":\"dcf0e4cd-c5e5-4129-a80f-1cd05790def0\"}]},\"type\":\"ConnectorPlacement.EquallySpacedConnector\",\"uuid\":\"218acaa3-d922-4814-a102-8c4fe12f2e05\"}],\"packageUris\":[\"http://schema.mathworks.com/mf0/Connector/R2020b\"],\"version\":\"1.0\"}"
  bst_set : Subsystem
      settings: PortSchema="{\"entries\":[{\"content\":{\"headerSize\":26,\"margin\":15,\"minimumSpacing\":25,\"sides\":[{\"content\":{\"connectorIds\":[\"In1\"]},\"type\":\"ConnectorPlacement.EquallySpacedRectSide\",\"uuid\":\"b493315f-c6c8-42ab-8e4d-b8fe240af9dd\"},{\"content\":{\"connectorIds\":[\"Out1\"],\"side\":\"RIGHT\"},\"type\":\"ConnectorPlacement.EquallySpacedRectSide\",\"uuid\":\"94c0e42b-c474-4070-8a16-a26ac22942e6\"},{\"content\":{\"side\":\"TOP\"},\"type\":\"ConnectorPlacement.EquallySpacedRectSide\",\"uuid\":\"f9bc43e9-5c3a-451c-b434-9225c48927cc\"},{\"content\":{\"side\":\"BOTTOM\"},\"type\":\"ConnectorPlacement.EquallySpacedRectSide\",\"uuid\":\"561f7f4a-dd6b-4ca4-b56e-b79619c3d586\"}]},\"type\":\"ConnectorPlacement.EquallySpacedConnector\",\"uuid\":\"067458af-ee7c-44e6-8802-98d558b25815\"}],\"packageUris\":[\"http://schema.mathworks.com/mf0/Connector/R2020b\"],\"version\":\"1.0\"}"
  process_pet : Subsystem
      settings: PortSchema="{\"entries\":[{\"content\":{\"headerSize\":26,\"margin\":15,\"minimumSpacing\":25,\"sides\":[{\"content\":{\"connectorIds\":[\"In1\",\"In2\"]},\"type\":\"ConnectorPlacement.EquallySpacedRectSide\",\"uuid\":\"d9face5b-155e-4e83-95c0-d581b737b6e3\"},{\"content\":{\"connectorIds\":[\"Out1\",\"Out2\",\"Out3\"],\"side\":\"RIGHT\"},\"type\":\"ConnectorPlacement.EquallySpacedRectSide\",\"uuid\":\"f965be1f-1639-4140-b9ea-f5e9efbe4150\"},{\"content\":{\"side\":\"TOP\"},\"type\":\"ConnectorPlacement.EquallySpacedRectSide\",\"uuid\":\"7c9c4b2b-011c-4482-afab-b6e67025a5e2\"},{\"content\":{\"side\":\"BOTTOM\"},\"type\":\"ConnectorPlacement.EquallySpacedRectSide\",\"uuid\":\"15505563-3824-4220-9d23-0c354b74bef5\"}]},\"type\":\"ConnectorPlacement.EquallySpacedConnector\",\"uuid\":\"ec963004-117d-4f22-bb00-71f35201e6e2\"}],\"packageUris\":[\"http://schema.mathworks.com/mf0/Connector/R2020b\"],\"version\":\"1.0\"}"
  Bus Element Out1 : Outport  PortName=bst_call(@external)
  Bus Element Out3 : Outport  Port=2  PortName=GlobalData.GUI
  wires:
  ? -> bst_get/1(bst_get(@db))
  bst_set/1(bst_set(@db)) -> ?
  ? -> ?
  Anatomy/2(BstMriFile) -> process_pet/2(BstMriFile)

== system pet_integration_architecture/Dataset Server/bids dataset ==
  Bus Element Out1 : Outport  AllowServiceAccess=on  PortName=userConfigRemote

== system pet_integration_architecture/Dataset Server/brainstorm_db ==

== system pet_integration_architecture/Dataset Server/remoteConfig ==
  Bus Element Out1 : Outport  AllowServiceAccess=on  PortName=userConfigRemote

== system pet_integration_architecture/Dataset Server/sourceData ==
  Out Bus Element1 : Outport  PortName=local

== system pet_integration_architecture/Freesurfer//Brainsuite/Brainsuite ==

== system pet_integration_architecture/Freesurfer//Brainsuite/Freesurfer ==
  note: Remote Data
  Bus Element In1 : Inport  AllowServiceAccess=on  PortName=local.fs
  LORIS Data Ingestor : Subsystem  VariantControl=LORIS Data Ingestor
      settings: PortSchema="{\"entries\":[{\"content\":{\"headerSize\":26,\"margin\":15,\"minimumSpacing\":25,\"sides\":[{\"content\":{},\"type\":\"ConnectorPlacement.EquallySpacedRectSide\",\"uuid\":\"a3539b9a-22db-4da3-b271-35b287ced3a1\"},{\"content\":{\"side\":\"RIGHT\"},\"type\":\"ConnectorPlacement.EquallySpacedRectSide\",\"uuid\":\"72d9f298-5062-46d4-b3c5-f2fa85d7a7a6\"},{\"content\":{\"side\":\"TOP\"},\"type\":\"ConnectorPlacement.EquallySpacedRectSide\",\"uuid\":\"050469fd-3881-4b53-a813-94df038aa659\"}]},\"type\":\"ConnectorPlacement.EquallySpacedConnector\",\"uuid\":\"6db04dad-62f3-4987-a6a9-d236db4fe2a3\"}],\"packageUris\":[\"http://schema.mathworks.com/mf0/Connector/R2020b\"],\"version\":\"1.0\"}"
  Linux : Subsystem  VariantControl=true
      settings: PortSchema="{\"entries\":[{\"content\":{\"headerSize\":26,\"margin\":15,\"minimumSpacing\":25,\"sides\":[{\"content\":{},\"type\":\"ConnectorPlacement.EquallySpacedRectSide\",\"uuid\":\"911b8937-6523-479c-8943-03fc0840c002\"},{\"content\":{\"connectorIds\":[\"In1\"],\"side\":\"RIGHT\"},\"type\":\"ConnectorPlacement.EquallySpacedRectSide\",\"uuid\":\"173af9ff-b0ec-4d9e-90c2-c5784cb94bd8\"},{\"content\":{\"side\":\"TOP\"},\"type\":\"ConnectorPlacement.EquallySpacedRectSide\",\"uuid\":\"a780b71c-d451-4700-b588-b61701b38ff2\"}]},\"type\":\"ConnectorPlacement.EquallySpacedConnector\",\"uuid\":\"e570ec77-32ef-4956-af7c-5098888363b1\"}],\"packageUris\":[\"http://schema.mathworks.com/mf0/Connector/R2020b\"],\"version\":\"1.0\"}"
  Windows : Subsystem  VariantControl=false
      settings: PortSchema="{\"entries\":[{\"content\":{\"headerSize\":26,\"margin\":15,\"minimumSpacing\":25,\"sides\":[{\"content\":{},\"type\":\"ConnectorPlacement.EquallySpacedRectSide\",\"uuid\":\"911b8937-6523-479c-8943-03fc0840c002\"},{\"content\":{\"connectorIds\":[\"In1\"],\"side\":\"RIGHT\"},\"type\":\"ConnectorPlacement.EquallySpacedRectSide\",\"uuid\":\"173af9ff-b0ec-4d9e-90c2-c5784cb94bd8\"},{\"content\":{\"side\":\"TOP\"},\"type\":\"ConnectorPlacement.EquallySpacedRectSide\",\"uuid\":\"a780b71c-d451-4700-b588-b61701b38ff2\"}]},\"type\":\"ConnectorPlacement.EquallySpacedConnector\",\"uuid\":\"e570ec77-32ef-4956-af7c-5098888363b1\"}],\"packageUris\":[\"http://schema.mathworks.com/mf0/Connector/R2020b\"],\"version\":\"1.0\"}"
  gitClone Brainstorm : Subsystem  VariantControl=gitClone Brainstorm
      settings: PortSchema="{\"entries\":[{\"content\":{\"headerSize\":26,\"margin\":15,\"minimumSpacing\":25,\"sides\":[{\"content\":{},\"type\":\"ConnectorPlacement.EquallySpacedRectSide\",\"uuid\":\"a3539b9a-22db-4da3-b271-35b287ced3a1\"},{\"content\":{\"connectorIds\":[\"In1\"],\"side\":\"RIGHT\"},\"type\":\"ConnectorPlacement.EquallySpacedRectSide\",\"uuid\":\"72d9f298-5062-46d4-b3c5-f2fa85d7a7a6\"},{\"content\":{\"side\":\"TOP\"},\"type\":\"ConnectorPlacement.EquallySpacedRectSide\",\"uuid\":\"050469fd-3881-4b53-a813-94df038aa659\"}]},\"type\":\"ConnectorPlacement.EquallySpacedConnector\",\"uuid\":\"6db04dad-62f3-4987-a6a9-d236db4fe2a3\"}],\"packageUris\":[\"http://schema.mathworks.com/mf0/Connector/R2020b\"],\"version\":\"1.0\"}"
